simulink model "lab3_2_model"  (R2014b)
settings: Solver=ode45  StartTime=0.0  StopTime=10.0  RelTol=1e-3
libraries: simulink x1
settings Model: Creator=NoteIP110  LastModifiedBy=NoteIP110

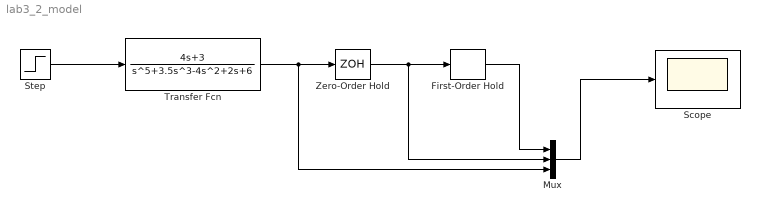
== system lab3_2_model ==
  First-Order Hold : simulink/Discrete/First-Order Hold  DisableCoverage=on  Ts=0.3
  Mux : Mux  Inputs=3
  Scope : Scope
      settings: ShowLegends=on
  Step : Step  SampleTime=0
  Transfer Fcn : TransferFcn  Numerator=[4 3]  Denominator=[1 0 3.5 -4 2 6]
  Zero-Order Hold : ZeroOrderHold  SampleTime=0.3
  wires:
  Step/1 -> Transfer Fcn/1
  Zero-Order Hold/1 -> Mux/2, First-Order Hold/1
  Transfer Fcn/1 -> Mux/3, Zero-Order Hold/1
  Mux/1 -> Scope/1
  First-Order Hold/1 -> Mux/1
